simulink model "a1_Conventional_IFPR_SYNINER_EUROPE_5s_C_18b"  (R2018b)
settings: Solver=VariableStepAuto  StartTime=0  StopTime=80  RelTol=1e-3
values from neighbouring files (symbols this model uses):
  ci = 0    [calc_nadir_IBFPR_SI.m]    (also in calc_variables_a1Ta.m = 1)
  E_load = 150    [a1_Conventional_mechlimit_EUR.m]    (also in calc_criticaltime.m; calc_nadir_IBFPR_SI.m; calc_variables_a1Ta.m; power_reserve.m)
  H = Ek/Sb    (= 0.375)    [a1_Conventional_mechlimit_EUR.m]    (also in calc_criticaltime.m = 3.75; calc_nadir_IBFPR_SI.m = 1.035; calc_variables_a1Ta.m = 2.25; power_reserve.m = 3.75)
  H_wt = 4.19    [calc_nadir_IBFPR_SI.m]    (also in calc_variables_a1Ta.m)
  J = 3.56    [calc_nadir_IBFPR_SI.m]    (also in calc_variables_a1Ta.m)
  Ki = 10    [calc_nadir_IBFPR_SI.m]    (also in calc_variables_a1Ta.m)
  n_wt = P_re*share_wt/(1.5e-3)    (= 61200)    [calc_nadir_IBFPR_SI.m]    (also in calc_variables_a1Ta.m = 48000)
  P_wt = P_re*share_wt    (= 91.8)    [calc_nadir_IBFPR_SI.m]    (also in calc_variables_a1Ta.m = 72)
  Sb = 200    [a1_Conventional_mechlimit_EUR.m]    (also in calc_criticaltime.m; calc_nadir_IBFPR_SI.m = 166.666666667; calc_variables_a1Ta.m = 166.666666667; power_reserve.m)
  T_1 = data1(2)    [a1_Conventional_mechlimit_EUR.m]    (also in calc_criticaltime.m; calc_nadir_IBFPR_SI.m; calc_variables_a1Ta.m; power_reserve.m)
  T_2 = data1(3)    [a1_Conventional_mechlimit_EUR.m]    (also in calc_criticaltime.m; calc_nadir_IBFPR_SI.m; calc_variables_a1Ta.m; power_reserve.m)
  T_3 = data1(4)    [a1_Conventional_mechlimit_EUR.m]    (also in calc_criticaltime.m; calc_nadir_IBFPR_SI.m; calc_variables_a1Ta.m; power_reserve.m)
  T_4 = data1(5)    [a1_Conventional_mechlimit_EUR.m]    (also in calc_criticaltime.m; calc_nadir_IBFPR_SI.m; calc_variables_a1Ta.m; power_reserve.m)
  T_wt = 1    [calc_nadir_IBFPR_SI.m]    (also in calc_variables_a1Ta.m)
  un = 0.02    [calc_nadir_IBFPR_SI.m]    (also in calc_variables_a1Ta.m)
undefined symbols (not defined in the file or in its folder): cfp
libraries: simulink x1
settings Model: Creator=estuser04  LastModifiedBy=Alejandro
settings SolverCC: AlgebraicLoopSolver=LineSearch

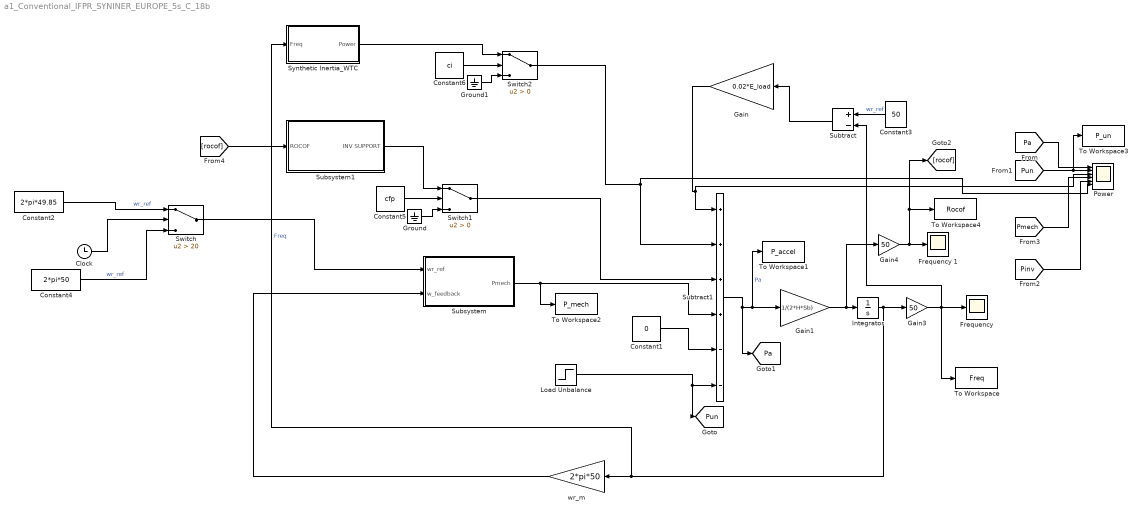
== system a1_Conventional_IFPR_SYNINER_EUROPE_5s_C_18b ==
  Clock : Clock
  Constant1 : Constant  Value=0
  Constant2 : Constant  Value=2*pi*49.85
  Constant3 : Constant  Value=50
  Constant4 : Constant  Value=2*pi*50
  Constant5 : Constant  Value=cfp
  Constant6 : Constant  Value=ci
  "Frequency " : Scope
  Frequency 1 : Scope
  Gain : Gain  Gain=0.02*E_load
  Gain1 : Gain  Gain=1/(2*H*Sb)
  Gain3 : Gain  Gain=50
  Gain4 : Gain  Gain=50
  Ground : Ground
  Ground1 : Ground
  Integrator : Integrator  InitialCondition=1
  Load Unbalance : Step  Time=0  After=E_load*un  SampleTime=0
  Power : Scope  NumInputPorts=6
  Subsystem : Subsystem
  Subsystem1 : Subsystem
  Subtract : Sum  Inputs=+-
  Subtract1 : Sum  Inputs=++++--
  Switch : Switch  Criteria=u2 > Threshold  Threshold=20
  Switch1 : Switch  Criteria=u2 > Threshold
  Switch2 : Switch  Criteria=u2 > Threshold
  "Synthetic Inertia_WTC " : Subsystem
  To Workspace : ToWorkspace  VariableName=Freq  SaveFormat=Timeseries  SampleTime=-1
  To Workspace1 : ToWorkspace  VariableName=P_accel  SaveFormat=Timeseries  SampleTime=-1
  To Workspace2 : ToWorkspace  VariableName=P_mech  SaveFormat=Timeseries  SampleTime=-1
  To Workspace3 : ToWorkspace  VariableName=P_un  SaveFormat=Timeseries  SampleTime=-1
  To Workspace4 : ToWorkspace  VariableName=Rocof  SaveFormat=Timeseries  SampleTime=-1
  "wr_m " : Gain  Gain=2*pi*50
  tag scope: Pa=global, Pun=global
  wires:
  Integrator/1 -> Gain3/1, "Synthetic Inertia_WTC "/1(Freq), "wr_m "/1  "Freq"
  Subtract1/1 -> [Pa], To Workspace1/1, Gain1/1  "Pa"
  Constant1/1 -> Subtract1/5
  Constant2/1 -> Switch/1  "wr_ref"
  "wr_m "/1 -> Subsystem/2(w_feedback)
  Subsystem/1(Pmech) -> Subtract1/4, To Workspace2/1
  [Pa] -> Power/1
  [Pun] -> To Workspace3/1, Power/2
  [Pmech] -> Power/4
  Gain1/1 -> Gain4/1, Integrator/1
  Gain4/1 -> [rocof], To Workspace4/1, Frequency 1/1
  Constant3/1 -> Subtract/1  "wr_ref"
  Subtract/1 -> Gain/1
  Gain3/1 -> Subtract/2, To Workspace/1, "Frequency "/1
  Gain/1 -> Subtract1/1, Power/3
  Load Unbalance/1 -> Subtract1/6, [Pun]
  Constant4/1 -> Switch/3  "wr_ref"
  Clock/1 -> Switch/2
  Switch/1 -> Subsystem/1(wr_ref)
  [Pinv] -> Power/5
  Subsystem1/1(INV SUPPORT) -> Switch1/1
  Ground/1 -> Switch1/3
  Constant5/1 -> Switch1/2
  Switch1/1 -> Subtract1/3
  [rocof] -> Subsystem1/1(ROCOF)
  Switch2/1 -> Subtract1/2, Power/6
  "Synthetic Inertia_WTC "/1("Power ") -> Switch2/1
  Constant6/1 -> Switch2/2
  Ground1/1 -> Switch2/3

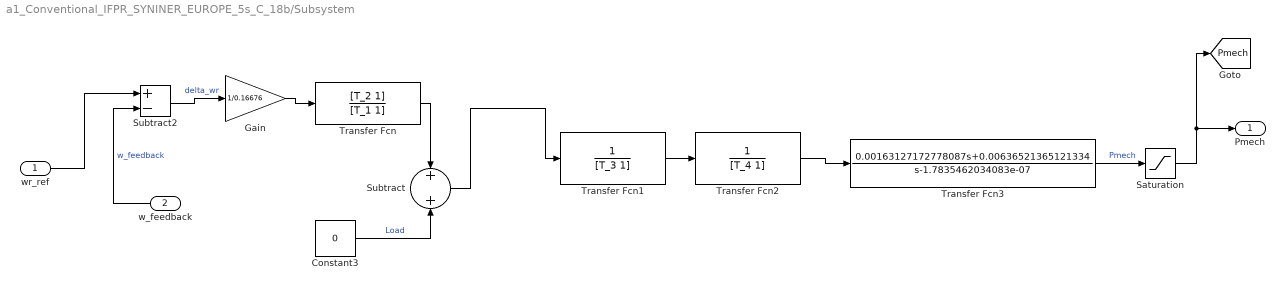
== system a1_Conventional_IFPR_SYNINER_EUROPE_5s_C_18b/Subsystem ==
  wr_ref : Inport
  w_feedback : Inport  Port=2
  Constant3 : Constant  Value=0
  Gain : Gain  Gain=1/0.16676
  Saturation : Saturate  UpperLimit=un*E_load  LowerLimit=0
  Subtract : Sum
  Subtract2 : Sum  Inputs=+-
  Transfer Fcn : TransferFcn  Numerator=[T_2 1]  Denominator=[T_1 1]
  Transfer Fcn1 : TransferFcn  Denominator=[T_3 1]
  Transfer Fcn2 : TransferFcn  Denominator=[T_4 1]
  Transfer Fcn3 : TransferFcn  Numerator=[0.00163127172778087 0.00636521365121334]  Denominator=[1 -1.7835462034083e-07]
  Pmech : Outport
  tag scope: Pmech=global
  wires:
  Constant3/1 -> Subtract/2  "Load"
  Transfer Fcn/1 -> Subtract/1
  Gain/1 -> Transfer Fcn/1
  Transfer Fcn2/1 -> Transfer Fcn3/1
  w_feedback/1 -> Subtract2/2  "w_feedback"
  Transfer Fcn1/1 -> Transfer Fcn2/1
  wr_ref/1 -> Subtract2/1
  Transfer Fcn3/1 -> Saturation/1  "Pmech"
  Subtract2/1 -> Gain/1  "delta_wr"
  Subtract/1 -> Transfer Fcn1/1
  Saturation/1 -> [Pmech], Pmech/1

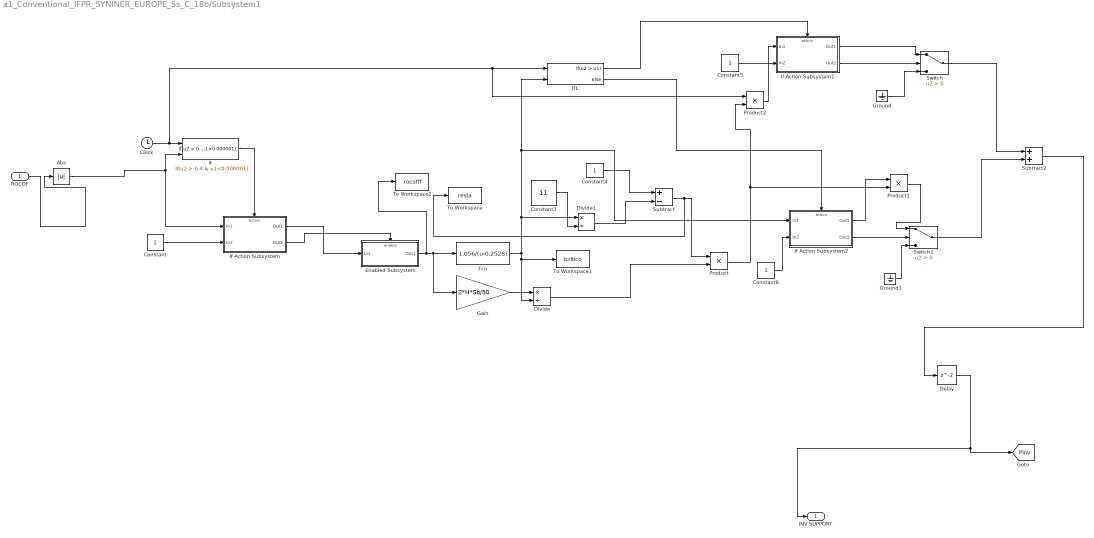
== system a1_Conventional_IFPR_SYNINER_EUROPE_5s_C_18b/Subsystem1 ==
  ROCOF : Inport
  Abs : Abs
  Clock : Clock
  Constant{,4..6} (4 alike) : Constant
  Constant3 : Constant  Value=11
  Delay : Delay  SampleTime=0.001
  Divide : Product  Inputs=*/
  Divide1 : Product  Inputs=*/
  Enabled Subsystem : Subsystem  TreatAsAtomicUnit=on
  Fcn : Fcn  Expr=1.056/(u-0.2528)
  Gain : Gain  Gain=2*H*Sb/50
  Ground : Ground
  Ground1 : Ground
  If : If  NumInputs=2  IfExpression=u2 > 0.4 & u1<0.000001  ShowElse=off
  If Action Subsystem : Subsystem  TreatAsAtomicUnit=on
  If Action Subsystem1 : Subsystem  TreatAsAtomicUnit=on
  If Action Subsystem2 : Subsystem  TreatAsAtomicUnit=on
  If1 : If  NumInputs=2  IfExpression=u2 > u1
  Product : Product
  Product1 : Product
  Product2 : Product
  Subtract : Sum  Inputs=+-
  Subtract2 : Sum
  Switch : Switch  Criteria=u2 > Threshold
  Switch1 : Switch  Criteria=u2 > Threshold
  To Workspace : ToWorkspace  VariableName=resta  SaveFormat=Timeseries  SampleTime=-1
  To Workspace1 : ToWorkspace  VariableName=tcritico  SaveFormat=Timeseries  SampleTime=-1
  To Workspace2 : ToWorkspace  VariableName=rocofff  SaveFormat=Timeseries  SampleTime=-1
  INV SUPPORT : Outport
  tag scope: Pinv=global
  wires:
  Switch1/1 -> Subtract2/2
  If Action Subsystem2/2(Out2) -> Switch1/2
  Divide/1 -> Product/2
  Product/1 -> Product1/2, Product2/2
  Constant4/1 -> Subtract/1
  Fcn/1 -> Divide/2, To Workspace1/1, If Action Subsystem2/1(In1), If1/2, Divide1/1
  If Action Subsystem/2(Out2) -> Enabled Subsystem/Enable
  Clock/1 -> Product2/1, If1/1, If/1
  Ground/1 -> Switch/3
  Divide1/1 -> Subtract/2
  Constant3/1 -> Divide1/2
  Enabled Subsystem/1(Out1) -> To Workspace2/1, Gain/1, Fcn/1
  If Action Subsystem/1(Out1) -> Enabled Subsystem/1(In1)
  Subtract/1 -> To Workspace/1, Product/1
  If Action Subsystem1/2(Out2) -> Switch/2
  If1/1 -> If Action Subsystem1/Action
  Subtract2/1 -> Delay/1
  Gain/1 -> Divide/1
  Ground1/1 -> Switch1/3
  If Action Subsystem2/1(Out1) -> Product1/1
  Product1/1 -> Switch1/1
  If Action Subsystem1/1(Out1) -> Switch/1
  Constant6/1 -> If Action Subsystem2/2(In2)
  Constant5/1 -> If Action Subsystem1/2(In2)
  Switch/1 -> Subtract2/1
  Constant/1 -> If Action Subsystem/2(In2)
  Abs/1 -> If Action Subsystem/1(In1), If/2
  If1/2 -> If Action Subsystem2/Action
  Product2/1 -> If Action Subsystem1/1(In1)
  Delay/1 -> [Pinv], INV SUPPORT/1
  If/1 -> If Action Subsystem/Action
  ROCOF/1 -> Abs/1

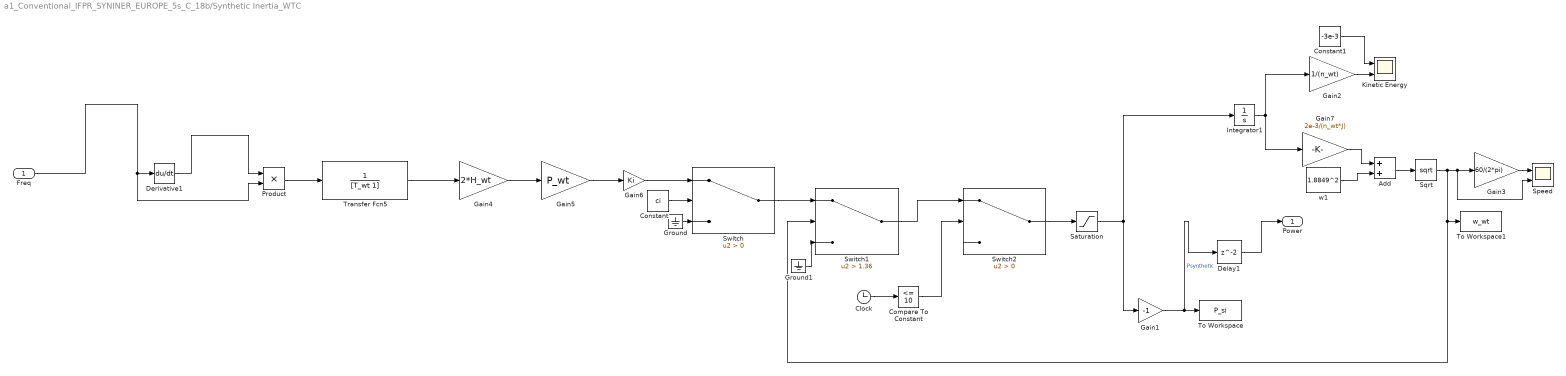
== system a1_Conventional_IFPR_SYNINER_EUROPE_5s_C_18b/Synthetic Inertia_WTC  ==
  Freq : Inport
  Add : Sum
  Clock : Clock
  Compare To Constant : simulink/Logic and Bit Operations/Compare To Constant  relop=<=  const=10  OutDataTypeStr=boolean
  Constant : Constant  Value=ci
  Constant1 : Constant  Value=-3e-3
  Delay1 : Delay  SampleTime=0.001
  Derivative1 : Derivative
  Gain1 : Gain  Gain=-1
  Gain2 : Gain  Gain=1/(n_wt)
  Gain3 : Gain  Gain=60/(2*pi)
  Gain4 : Gain  Gain=2*H_wt
  Gain5 : Gain  Gain=P_wt
  Gain6 : Gain  Gain=Ki
  Gain7 : Gain  Gain=2e-3/(n_wt*J)
  Ground : Ground
  Ground1 : Ground
  Integrator1 : Integrator
  "Kinetic Energy " : Scope  NumInputPorts=2
  Product : Product
  Saturation : Saturate  UpperLimit=0  LowerLimit=-P_wt*0.10
  "Speed " : Scope  NumInputPorts=2
  Sqrt : Sqrt  SaturateOnIntegerOverflow=on
  Switch : Switch  Criteria=u2 > Threshold
  Switch1 : Switch  Criteria=u2 > Threshold  Threshold=1.36
  Switch2 : Switch  Criteria=u2 > Threshold
  To Workspace : ToWorkspace  VariableName=P_si  SaveFormat=Timeseries  SampleTime=-1
  To Workspace1 : ToWorkspace  VariableName=w_wt  SaveFormat=Timeseries  SampleTime=-1
  Transfer Fcn5 : TransferFcn  Denominator=[T_wt 1]
  w1 : Constant  Value=1.8849^2
  "Power " : Outport
  wires:
  Gain5/1 -> Gain6/1
  Switch/1 -> Switch1/1
  Gain7/1 -> Add/1
  Gain4/1 -> Gain5/1
  Add/1 -> Sqrt/1
  w1/1 -> Add/2
  Product/1 -> Transfer Fcn5/1
  Transfer Fcn5/1 -> Gain4/1
  Constant/1 -> Switch/2
  Integrator1/1 -> Gain7/1, Gain2/1
  Gain6/1 -> Switch/1
  Ground/1 -> Switch/3
  Gain1/1 -> Delay1/1, To Workspace/1  "Psynthetic"
  Switch1/1 -> Switch2/1
  Sqrt/1 -> Switch1/2, To Workspace1/1, "Speed "/2, Gain3/1
  Ground1/1 -> Switch1/3
  Gain2/1 -> "Kinetic Energy "/2
  Constant1/1 -> "Kinetic Energy "/1
  Saturation/1 -> Gain1/1, Integrator1/1
  Derivative1/1 -> Product/1
  Gain3/1 -> "Speed "/1
  Clock/1 -> Compare To Constant/1
  Compare To Constant/1 -> Switch2/2
  Switch2/1 -> Saturation/1
  Freq/1 -> Product/2, Derivative1/1
  Delay1/1 -> "Power "/1

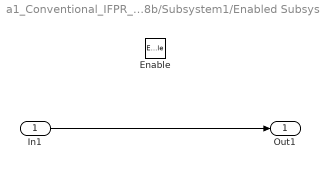
== system a1_Conventional_IFPR_SYNINER_EUROPE_5s_C_18b/Subsystem1/Enabled Subsystem ==
  In1 : Inport
  Enable : EnablePort
  Out1 : Outport  InitialOutput=1e-20
  wires:
  In1/1 -> Out1/1

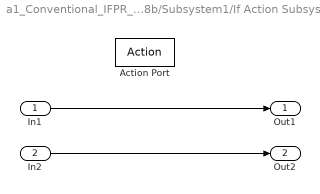
== system a1_Conventional_IFPR_SYNINER_EUROPE_5s_C_18b/Subsystem1/If Action Subsystem ==
  In1 : Inport
  In2 : Inport  Port=2
  Action Port : ActionPort
  Out1 : Outport
  Out2 : Outport  Port=2
  wires:
  In1/1 -> Out1/1
  In2/1 -> Out2/1

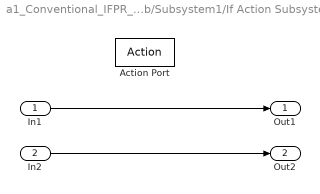
== system a1_Conventional_IFPR_SYNINER_EUROPE_5s_C_18b/Subsystem1/If Action Subsystem1 ==
  In1 : Inport
  In2 : Inport  Port=2
  Action Port : ActionPort
  Out1 : Outport  OutputWhenDisabled=reset  InitialOutput=0
  Out2 : Outport  Port=2  OutputWhenDisabled=reset  InitialOutput=0
  wires:
  In1/1 -> Out1/1
  In2/1 -> Out2/1

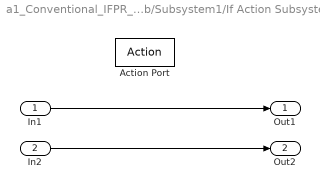
== system a1_Conventional_IFPR_SYNINER_EUROPE_5s_C_18b/Subsystem1/If Action Subsystem2 ==
  In1 : Inport
  In2 : Inport  Port=2
  Action Port : ActionPort
  Out1 : Outport  OutputWhenDisabled=reset  InitialOutput=0
  Out2 : Outport  Port=2  InitialOutput=0
  wires:
  In1/1 -> Out1/1
  In2/1 -> Out2/1
